simulink model "RIP_SMLThoang"  (R2020b)
settings: Solver=FixedStepAuto  StartTime=0.0  StopTime=20  FixedStep=0.01  RelTol=1e-3
values from neighbouring files (symbols this model uses):
  kd1 = par(bestchrom,3)-100    [PID_GA.m]    (also in test_PID.m = 0.35; thong_so_dieu_khien_RIP1.m = 0)
  kd2 = par(bestchrom,6)-100    [PID_GA.m]    (also in test_PID.m = 3.9; thong_so_dieu_khien_RIP1.m = 0)
  ki1 = par(bestchrom,2)-100    [PID_GA.m]    (also in thong_so_dieu_khien_RIP1.m = 0)
  ki2 = par(bestchrom,5)-100    [PID_GA.m]    (also in thong_so_dieu_khien_RIP1.m = 0)
  kp1 = par(bestchrom,1)-100    [PID_GA.m]    (also in test_PID.m = 0.88; thong_so_dieu_khien_RIP1.m = 50)
  kp2 = par(bestchrom,4)-100    [PID_GA.m]    (also in test_PID.m = 46; thong_so_dieu_khien_RIP1.m = 7)
  x1_init = 0.1    [PID_GA.m]    (also in thong_so_dieu_khien_RIP.m; thong_so_dieu_khien_RIP1.m = 0.314159265359)
  x2_init = 0    [PID_GA.m]    (also in thong_so_dieu_khien_RIP.m = -0.1; thong_so_dieu_khien_RIP1.m = 0.157079632679)
  x3_init = -0.1    [PID_GA.m]    (also in thong_so_dieu_khien_RIP.m = 0; thong_so_dieu_khien_RIP1.m = 0.01)
  x4_init = 0    [PID_GA.m]    (also in thong_so_dieu_khien_RIP.m; thong_so_dieu_khien_RIP1.m = 0.1)
undefined symbols (not defined in the file or in its folder): DiscIntNeverNeededParam
libraries: simulink x2
settings Model: Creator=OS  LastModifiedBy=OS

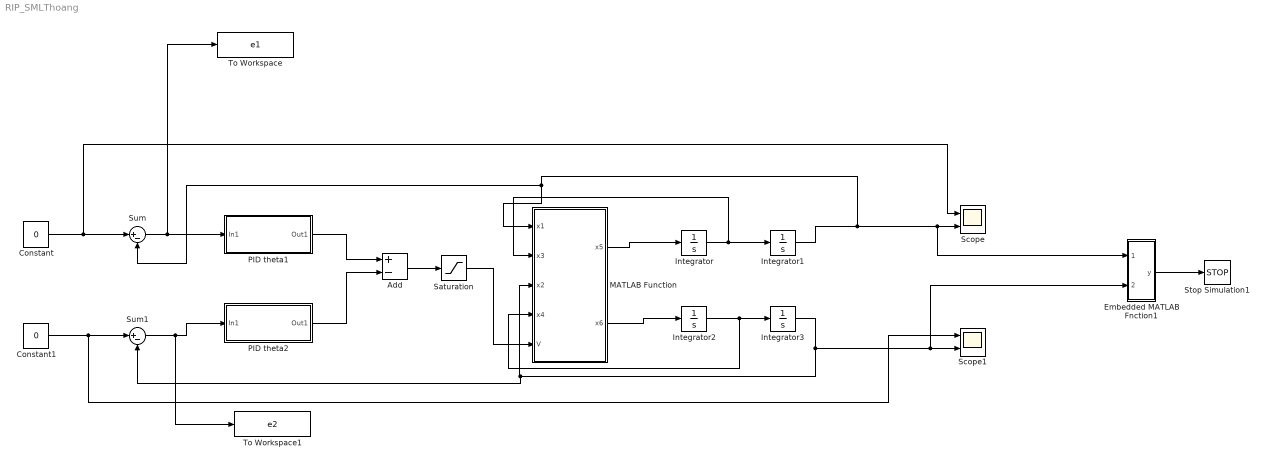
== system RIP_SMLThoang ==
  Add : Sum  Inputs=+-
  Constant : Constant  Value=0
  Constant1 : Constant  Value=0
  Embedded MATLAB Fnction1 : MATLAB Function  TreatAsAtomicUnit=on
  Integrator : Integrator  InitialCondition=x3_init
  Integrator1 : Integrator  InitialCondition=x1_init
  Integrator2 : Integrator  InitialCondition=x4_init
  Integrator3 : Integrator  InitialCondition=x2_init
  MATLAB Function : MATLAB Function  TreatAsAtomicUnit=on
  PID theta1 : Subsystem
  PID theta2 : Subsystem
  Saturation : Saturate  UpperLimit=11  LowerLimit=-11
  Scope : Scope  NumInputPorts=2
  Scope1 : Scope  NumInputPorts=2
  Stop Simulation1 : Stop
  Sum : Sum  Inputs=|+-
  Sum1 : Sum  Inputs=|+-
  To Workspace : ToWorkspace  VariableName=e1  SampleTime=0.01
  To Workspace1 : ToWorkspace  VariableName=e2  SampleTime=0.01
  wires:
  Constant1/1 -> Scope1/1, Sum1/1
  Integrator3/1 -> Embedded MATLAB Fnction1/2(e2), Scope1/2, Sum1/2, MATLAB Function/3(x2)
  Add/1 -> Saturation/1
  Constant/1 -> Scope/1, Sum/1
  Integrator1/1 -> MATLAB Function/1(x1), Sum/2, Embedded MATLAB Fnction1/1(e1), Scope/2
  PID theta2/1(Out1) -> Add/2
  Sum/1 -> To Workspace/1, PID theta1/1(In1)
  Saturation/1 -> MATLAB Function/5(V)
  MATLAB Function/2(x6) -> Integrator2/1
  MATLAB Function/1(x5) -> Integrator/1
  Sum1/1 -> To Workspace1/1, PID theta2/1(In1)
  Integrator/1 -> MATLAB Function/2(x3), Integrator1/1
  PID theta1/1(Out1) -> Add/1
  Integrator2/1 -> MATLAB Function/4(x4), Integrator3/1
  Embedded MATLAB Fnction1/1(y) -> Stop Simulation1/1

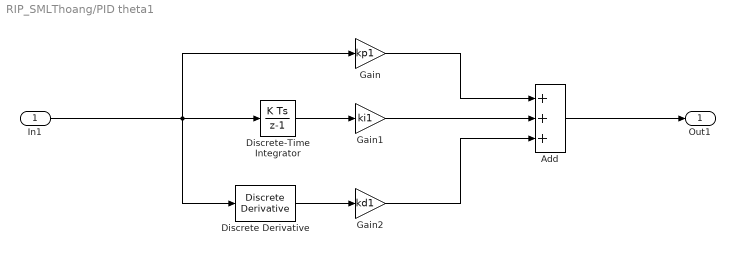
== system RIP_SMLThoang/PID theta1 ==
  In1 : Inport
  Add : Sum  Inputs=+++
  Discrete Derivative : simulink/Discrete/Discrete Derivative  gainval=1.0  ICPrevScaledInput=0.0  OutMin=[]  OutMax=[]  OutDataType=fixdt(1, 16)  OutScaling=2^-10  DoSatur=off
      link override TSamp: TsampMathImp=Offline Scaling Adjustment
  Discrete-Time Integrator : DiscreteIntegrator  SampleTime=-1  ICPrevOutput=DiscIntNeverNeededParam  ICPrevScaledInput=DiscIntNeverNeededParam
  Gain : Gain  Gain=kp1
  Gain1 : Gain  Gain=ki1
  Gain2 : Gain  Gain=kd1
  Out1 : Outport
  wires:
  Discrete Derivative/1 -> Gain2/1
  Discrete-Time Integrator/1 -> Gain1/1
  Gain/1 -> Add/1
  Gain1/1 -> Add/2
  Gain2/1 -> Add/3
  Add/1 -> Out1/1
  In1/1 -> Gain/1, Discrete Derivative/1, Discrete-Time Integrator/1

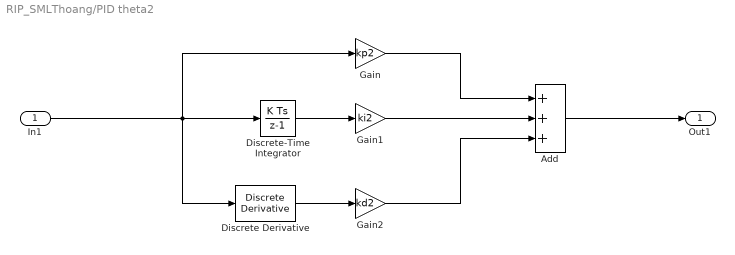
== system RIP_SMLThoang/PID theta2 ==
  In1 : Inport
  Add : Sum  Inputs=+++
  Discrete Derivative : simulink/Discrete/Discrete Derivative  gainval=1.0  ICPrevScaledInput=0.0  OutMin=[]  OutMax=[]  OutDataType=fixdt(1, 16)  OutScaling=2^-10  DoSatur=off
      link override TSamp: TsampMathImp=Offline Scaling Adjustment
  Discrete-Time Integrator : DiscreteIntegrator  SampleTime=-1  ICPrevOutput=DiscIntNeverNeededParam  ICPrevScaledInput=DiscIntNeverNeededParam
  Gain : Gain  Gain=kp2
  Gain1 : Gain  Gain=ki2
  Gain2 : Gain  Gain=kd2
  Out1 : Outport
  wires:
  Discrete Derivative/1 -> Gain2/1
  Discrete-Time Integrator/1 -> Gain1/1
  Gain/1 -> Add/1
  Gain1/1 -> Add/2
  Gain2/1 -> Add/3
  Add/1 -> Out1/1
  In1/1 -> Gain/1, Discrete Derivative/1, Discrete-Time Integrator/1

== matlab function RIP_SMLThoang/Embedded MATLAB Fnction1 ==
  data: e1 input; y output; e2 input
function y = fcn(e1,e2)
if (abs(e1)>(3))||(abs(e2)>(3))
    y=1;
else
    y=0;
end

== matlab function RIP_SMLThoang/MATLAB Function ==
  data: x1 input; x3 input; x5 output; x2 input; x4 input; V input; x6 output
function [x5,x6] = fcn(x1,x3,x2,x4,V)
% Thông số của hệ thống 
Kt = 0.07;  % Hằng số momen-xoắn của động cơ 
Kb = 0.07;  % Hằng số điện áp cảm ứng 
mp = 0.0319;  % Khối lượng của pendulum 
Lp = 0.1572;  % Chiều dài của pendulum 
Lr = 0.1370;  % Chiều dài của arm 
Jr = 0.008591;
Cm = 0.006408; 
Jp = 0.000217;
Bp = 0.001;  % Hệ số cản của pendulum
Rm = 1.7;  % Điện trở của động cơ 
Jm = 2.52e-5;  % Hằng số momen quán tính của động cơ 
g = 9.81 ;
x5 =-(2*Cm*Jp*Rm*x3 - 2*Kt*Lp^2*V*mp - 2*Jp*Kt*V + 2*Jp*Kb*Kt*x3 + 2*Cm*Lp^2*Rm*mp*x3 + 2*Kb*Kt*Lp^2*mp*x3 + 2*Lp^3*Lr*Rm*mp^2*x4^2*sin(x2) + 2*Lp^4*Rm*mp^2*x3*x4*sin(2*x2) + 2*Bp*Lp*Lr*Rm*mp*x4*cos(x2) + 2*Jp*Lp^2*Rm*mp*x3*x4*sin(2*x2) - Lp^3*Lr*Rm*mp^2*x3^2*sin(2*x2)*cos(x2) - 2*Lp^2*Lr*Rm*g*mp^2*cos(x2)*sin(x2) + 2*Jp*Lp*Lr*Rm*mp*x4^2*sin(x2))/(2*Rm*(Jm*Jp + Jp*Jr + Lp^4*mp^2*sin(x2)^2 + Lp^2*Lr^2*mp^2 + Jm*Lp^2*mp + Jp*Lr^2*mp + Jr*Lp^2*mp + Jp*Lp^2*mp*sin(x2)^2 - Lp^2*Lr^2*mp^2*cos(x2)^2));
 
x6 =(2*Lp^3*Rm*g*mp^2*sin(x2)^3 - 2*Bp*Jr*Rm*x4 - 2*Bp*Lr^2*Rm*mp*x4 - 2*Bp*Jm*Rm*x4 + 2*Jm*Lp*Rm*g*mp*sin(x2) + 2*Jr*Lp*Rm*g*mp*sin(x2) + Jm*Lp^2*Rm*mp*x3^2*sin(2*x2) + Jr*Lp^2*Rm*mp*x3^2*sin(2*x2) + Lp^4*Rm*mp^2*x3^2*sin(2*x2)*sin(x2)^2 + 2*Lp*Lr^2*Rm*g*mp^2*sin(x2) - 2*Bp*Lp^2*Rm*mp*x4*sin(x2)^2 + 2*Kt*Lp*Lr*V*mp*cos(x2) + Lp^2*Lr^2*Rm*mp^2*x3^2*sin(2*x2) - 2*Cm*Lp*Lr*Rm*mp*x3*cos(x2) - 2*Kb*Kt*Lp*Lr*mp*x3*cos(x2) - 2*Lp^2*Lr^2*Rm*mp^2*x4^2*cos(x2)*sin(x2) - 2*Lp^3*Lr*Rm*mp^2*x3*x4*sin(2*x2)*cos(x2))/(2*Rm*(Jm*Jp + Jp*Jr + Lp^4*mp^2*sin(x2)^2 + Lp^2*Lr^2*mp^2 + Jm*Lp^2*mp + Jp*Lr^2*mp + Jr*Lp^2*mp + Jp*Lp^2*mp*sin(x2)^2 - Lp^2*Lr^2*mp^2*cos(x2)^2));
end
